simulink model "HITL_Plant_top"  (R2026a)
settings: Solver=VariableStepAuto  StopTime=inf
undefined symbols (not defined in the file): airspeed, ddx, ddy, ddz, dx, dy, dz, fractalcoef, gpsFreq, heartbeatFreq, m_to_mm, ms_to_cms, p, Payload, pitch, q, r, roll, SampleTime, uT_to_gauss, X, Y, yaw, Z
libraries: uavmavlinklib x9, simulink x4, px4MAVLinkBridgelib x2, aerolibatmos2 x1, sensorgpslib x1, robotcorelib x1, mspsensorlib x1
settings Model: DataDictionary=VTOLDynamicsData.sldd  SimulationMode=accelerator  Creator=The MathWorks, Inc.  LastModifiedBy=The MathWorks, Inc.
settings RTWCC: LargeConstantGeneration=WriteOnlyDNNConstantsToDataFiles

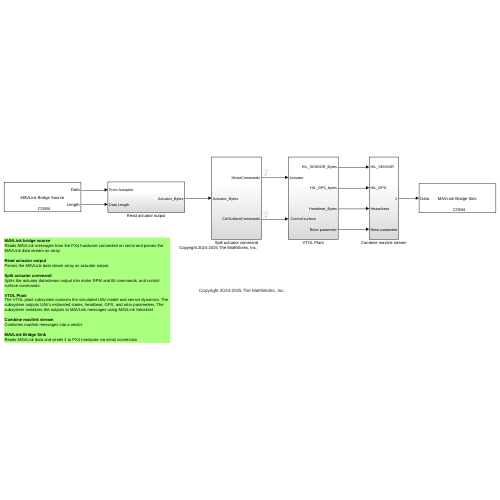
[thumbnail: Simulink's stored preview of the top-level diagram]
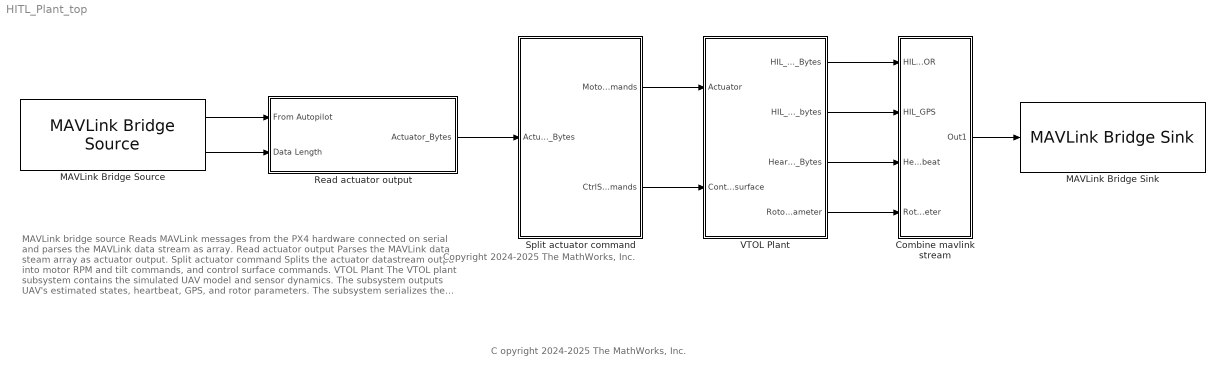
== system HITL_Plant_top ==
  note: MAVLink bridge source
      | Reads MAVLink messages from the PX4 hardware connected on serial and parses the MAVLink data stream as array.
      |
      | Read actuator output
      | Parses the MAVLink data steam array as actuator output.
      |
      | Split actuator command
      | Splits the actuator datastream output into motor RPM and tilt commands, and control surface commands.
      |
      | VTOL Plant
      | The VTOL plant subsystem contains the simulated UAV model and sensor dynamics. The subsystem outputs UAV's estimated states, heartbeat, GPS, and rotor parameters. The subsystem serializes the outputs to MAVLink messages using MAVLink Serializer
      |
      | Combine mavlink stream
      | Combines mavlink messages into a vector
      |
      | MAVLink Bridge Sink
      | Reads MAVLink data and sends it to PX4 hardware via serial connection
  note: C opyright 2024-2025 The MathWorks, Inc.
  note: Copyright 2024-2025 The MathWorks, Inc.
  Combine mavlink stream : Subsystem
  MAVLink Bridge Sink : px4MAVLinkBridgelib/MAVLink Bridge Sink  PixhawkSerialPorttemp=Specify manually  PixhawkSerialPortManually=COM4  FieldTable={ 'UDP', '127.0.0.1', '14550'; 'UDP', '127.0.0.1', '25000' }
  MAVLink Bridge Source : px4MAVLinkBridgelib/MAVLink Bridge Source  PixhawkSerialPorttemp=Specify manually  PixhawkSerialPortManually=COM4  dataLength=MAVLink_Input_Read_Size  FieldTable={ 'UDP', '127.0.0.1', '14550'; 'UDP', '127.0.0.1', '25000' }  SampleTime=SampleTime
  Read actuator output : Subsystem
  Split actuator command : Subsystem
  VTOL Plant : Subsystem
  wires:
  MAVLink Bridge Source/1 -> Read actuator output/1(From Autopilot)
  MAVLink Bridge Source/2 -> Read actuator output/2(Data Length)
  Read actuator output/1(Actuator_Bytes) -> Split actuator command/1(Actuator_Bytes)
  Split actuator command/1(MotorCommands) -> VTOL Plant/1(Actuator)
  Split actuator command/2(CtrlSurfaceCommands) -> VTOL Plant/2(" Control surface")
  Combine mavlink stream/1(Out1) -> MAVLink Bridge Sink/1
  VTOL Plant/2(HIL_GPS_bytes) -> Combine mavlink stream/2(HIL_GPS)
  VTOL Plant/3(Heartbeat_Bytes) -> Combine mavlink stream/3(Heaartbeat)
  VTOL Plant/4(Rotor parameter) -> Combine mavlink stream/4(Rotor parameter)
  VTOL Plant/1(HIL_SENSOR_Bytes) -> Combine mavlink stream/1(HIL_SENSOR)

== system HITL_Plant_top/Combine mavlink stream ==
  HIL_SENSOR : Inport
  HIL_GPS : Inport  Port=2
  Heaartbeat : Inport  Port=3
  Rotor parameter : Inport  Port=4
  Mux : Mux
  Out1 : Outport
  wires:
  Mux/1 -> Out1/1
  HIL_SENSOR/1 -> Mux/1
  HIL_GPS/1 -> Mux/2
  Heaartbeat/1 -> Mux/3
  Rotor parameter/1 -> Mux/4

== system HITL_Plant_top/Read actuator output ==
  From Autopilot : Inport
  Data Length : Inport  Port=2
  Constant : Constant  SampleTime=SampleTime
  Constant1 : Constant  Value=0  OutDataTypeStr=uint8  SampleTime=SampleTime
  Data Type Conversion : DataTypeConversion  OutDataTypeStr=double  SaturateOnIntegerOverflow=off  RndMeth=Floor
  Mux : Mux  Inputs=2
  Reshape : Reshape
  Selector : Selector  InputPortWidth=MAVLink_Input_Read_Size  IndexOptions=Starting and ending indices (port)  Indices=[1 3]  OutputSizes=1
  Switch : Switch  Criteria=u2 > Threshold  SaturateOnIntegerOverflow=off  InputSameDT=off
  Actuator_Bytes : Outport
  wires:
  Mux/1 -> Selector/2
  Constant/1 -> Mux/1
  Data Length/1 -> Data Type Conversion/1
  From Autopilot/1 -> Selector/1
  Switch/1 -> Reshape/1
  Selector/1 -> Switch/1
  Data Type Conversion/1 -> Switch/2, Mux/2
  Reshape/1 -> Actuator_Bytes/1
  Constant1/1 -> Switch/3

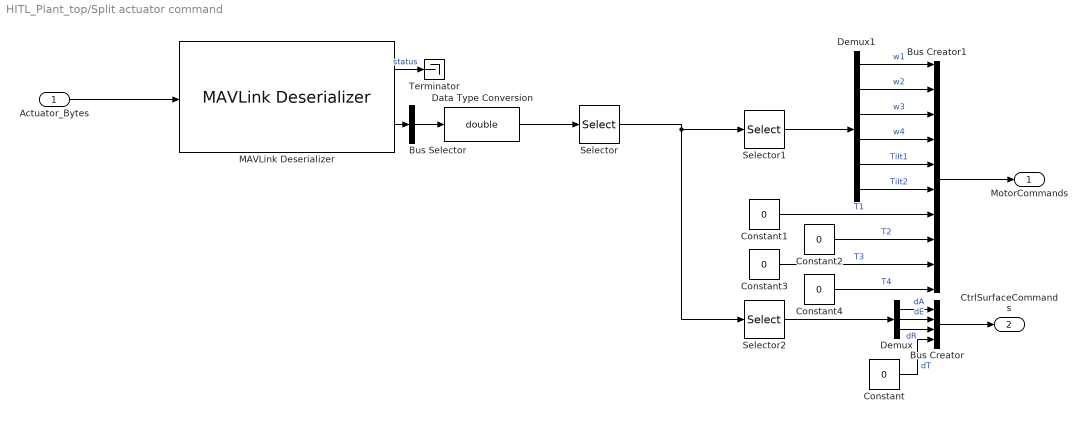
== system HITL_Plant_top/Split actuator command ==
  Actuator_Bytes : Inport
  Bus Creator : BusCreator  Inputs=4  OutDataTypeStr=Bus: FixedWingCtrlBus
  Bus Creator1 : BusCreator  Inputs=10  OutDataTypeStr=Bus: RotorCtrlBus
  Bus Selector : BusSelector  OutputSignals=Payload.controls  OutputAsBus=on
  Constant{,1..4} (5 alike) : Constant  Value=0
  Data Type Conversion : DataTypeConversion  OutDataTypeStr=double  SaturateOnIntegerOverflow=off  RndMeth=Floor
  Demux : Demux  Outputs=3
  Demux1 : Demux  Outputs=6
  MAVLink Deserializer : uavmavlinklib/MAVLink Deserializer  dialectSource=Select from standard MAVLink dialects  dialect=common.xml  dialectCustom=common.xml  version=2  messageType=HIL_ACTUATOR_CONTROLS  inputDataLength=off  SystemIDFilter=off  systemID=1  ComponentIDFilter=off  componentID=1  queueMsg=off  queueMsgSize=50  dropNum=off
  Selector : Selector  InputPortWidth=16  IndexOptions=Index vector (dialog)  Indices=[1:9]  OutputSizes=1
  Selector1 : Selector  InputPortWidth=9  IndexOptions=Index vector (dialog)  Indices=[1:6]  OutputSizes=1
  Selector2 : Selector  InputPortWidth=9  IndexOptions=Index vector (dialog)  Indices=[7:9]  OutputSizes=1
  Terminator : Terminator
  MotorCommands : Outport
  CtrlSurfaceCommands : Outport  Port=2
  wires:
  Actuator_Bytes/1 -> MAVLink Deserializer/1
  Bus Creator1/1 -> MotorCommands/1
  Demux/1 -> Bus Creator/1  "dA"
  Demux1/6 -> Bus Creator1/6  "Tilt2"
  Data Type Conversion/1 -> Selector/1
  Bus Creator/1 -> CtrlSurfaceCommands/1
  Demux1/1 -> Bus Creator1/1  "w1"
  Demux/2 -> Bus Creator/2  "dE"
  MAVLink Deserializer/2 -> Bus Selector/1
  Demux1/2 -> Bus Creator1/2  "w2"
  Demux1/5 -> Bus Creator1/5  "Tilt1"
  MAVLink Deserializer/1 -> Terminator/1  "status"
  Selector2/1 -> Demux/1
  Demux/3 -> Bus Creator/3  "dR"
  Demux1/3 -> Bus Creator1/3  "w3"
  Demux1/4 -> Bus Creator1/4  "w4"
  Bus Selector/1 -> Data Type Conversion/1
  Selector1/1 -> Demux1/1
  Selector/1 -> Selector2/1, Selector1/1
  Constant/1 -> Bus Creator/4  "dT"
  Constant1/1 -> Bus Creator1/7  "T1"
  Constant2/1 -> Bus Creator1/8  "T2"
  Constant3/1 -> Bus Creator1/9  "T3"
  Constant4/1 -> Bus Creator1/10  "T4"

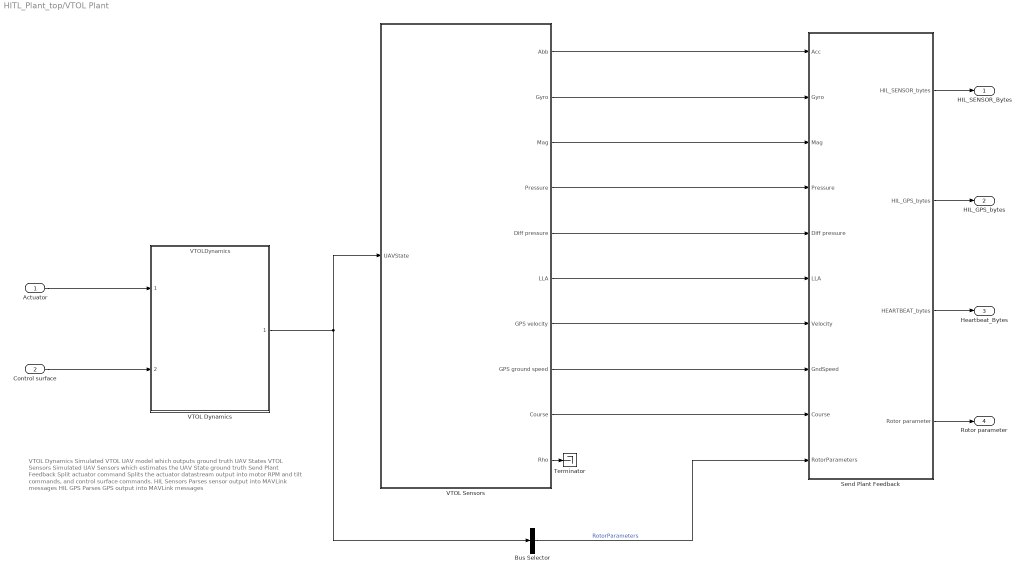
== system HITL_Plant_top/VTOL Plant ==
  note: VTOL Dynamics
      | Simulated VTOL UAV model which outputs ground truth UAV States
      |
      | VTOL Sensors
      | Simulated UAV Sensors which estimates the UAV State ground truth
      |
      | Send Plant Feedback
      | Split actuator command
      | Splits the actuator datastream output into motor RPM and tilt commands, and control surface commands.
      |
      | HIL Sensors
      | Parses sensor output into MAVLink messages
      |
      | HIL GPS
      | Parses GPS output into MAVLink messages
  Actuator : Inport
  " Control surface" : Inport  Port=2
  Bus Selector : BusSelector  OutputSignals=RotorParameters  OutputAsBus=on
  Send Plant Feedback : Subsystem
  Terminator : Terminator
  VTOL Dynamics : ModelReference  ModelNameDialog=VTOLDynamics  SimulationMode=Normal  ModelReferenceVersion=4.0
  VTOL Sensors : Subsystem
  HIL_SENSOR_Bytes : Outport
  HIL_GPS_bytes : Outport  Port=2
  Heartbeat_Bytes : Outport  Port=3
  Rotor parameter : Outport  Port=4
  wires:
  Actuator/1 -> VTOL Dynamics/1
  " Control surface"/1 -> VTOL Dynamics/2
  VTOL Dynamics/1 -> Bus Selector/1, VTOL Sensors/1(UAVState)
  VTOL Sensors/10(Rho) -> Terminator/1
  VTOL Sensors/1(Abb) -> Send Plant Feedback/1(Acc)
  VTOL Sensors/2(Gyro) -> Send Plant Feedback/2(Gyro)
  VTOL Sensors/3(Mag) -> Send Plant Feedback/3(Mag)
  VTOL Sensors/4(Pressure) -> Send Plant Feedback/4(Pressure)
  VTOL Sensors/5(Diff pressure) -> Send Plant Feedback/5(Diff pressure)
  VTOL Sensors/6(LLA) -> Send Plant Feedback/6(LLA)
  VTOL Sensors/7(GPS velocity) -> Send Plant Feedback/7(Velocity)
  VTOL Sensors/8(GPS ground speed) -> Send Plant Feedback/8(GndSpeed)
  VTOL Sensors/9(Course) -> Send Plant Feedback/9(Course)
  Bus Selector/1 -> Send Plant Feedback/10(RotorParameters)  "RotorParameters"
  Send Plant Feedback/1(HIL_SENSOR_bytes) -> HIL_SENSOR_Bytes/1
  Send Plant Feedback/2(HIL_GPS_bytes) -> HIL_GPS_bytes/1
  Send Plant Feedback/3(HEARTBEAT_bytes) -> Heartbeat_Bytes/1
  Send Plant Feedback/4(Rotor parameter) -> Rotor parameter/1

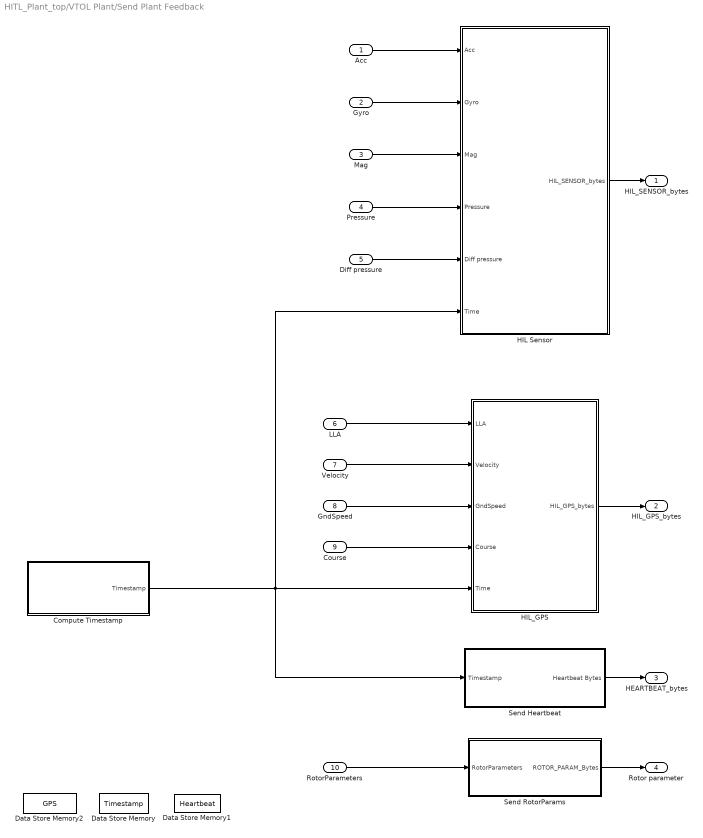
== system HITL_Plant_top/VTOL Plant/Send Plant Feedback ==
  Acc : Inport
  Gyro : Inport  Port=2
  Mag : Inport  Port=3
  Pressure : Inport  Port=4
  Diff pressure : Inport  Port=5
  LLA : Inport  Port=6
  Velocity : Inport  Port=7
  GndSpeed : Inport  Port=8
  Course : Inport  Port=9
  RotorParameters : Inport  Port=10
  Compute Timestamp : Subsystem  Priority=1
  Data Store Memory : DataStoreMemory  DataStoreName=Timestamp  WriteAfterWriteMsg=warning  ShowAdditionalParam=off
  Data Store Memory1 : DataStoreMemory  DataStoreName=Heartbeat  WriteAfterWriteMsg=warning  ShowAdditionalParam=off
  Data Store Memory2 : DataStoreMemory  DataStoreName=GPS  WriteAfterWriteMsg=warning  ShowAdditionalParam=off
  HIL Sensor : Subsystem  Priority=2
  HIL_GPS : Subsystem  Priority=3
  Send Heartbeat : Subsystem  Priority=4
  Send RotorParams : Subsystem  Priority=5
  HIL_SENSOR_bytes : Outport
  HIL_GPS_bytes : Outport  Port=2
  HEARTBEAT_bytes : Outport  Port=3
  Rotor parameter : Outport  Port=4
  wires:
  Send Heartbeat/1(Heartbeat Bytes) -> HEARTBEAT_bytes/1
  RotorParameters/1 -> Send RotorParams/1(RotorParameters)
  Mag/1 -> HIL Sensor/3(Mag)
  Send RotorParams/1(ROTOR_PARAM_Bytes) -> Rotor parameter/1
  Course/1 -> HIL_GPS/4(Course)
  Velocity/1 -> HIL_GPS/2(Velocity)
  Gyro/1 -> HIL Sensor/2(Gyro)
  GndSpeed/1 -> HIL_GPS/3(GndSpeed)
  Pressure/1 -> HIL Sensor/4(Pressure)
  HIL Sensor/1(HIL_SENSOR_bytes) -> HIL_SENSOR_bytes/1
  Acc/1 -> HIL Sensor/1(Acc)
  LLA/1 -> HIL_GPS/1(LLA)
  Diff pressure/1 -> HIL Sensor/5(Diff pressure)
  HIL_GPS/1(HIL_GPS_bytes) -> HIL_GPS_bytes/1
  Compute Timestamp/1(Timestamp) -> Send Heartbeat/1(Timestamp), HIL Sensor/6(Time), HIL_GPS/5(Time)

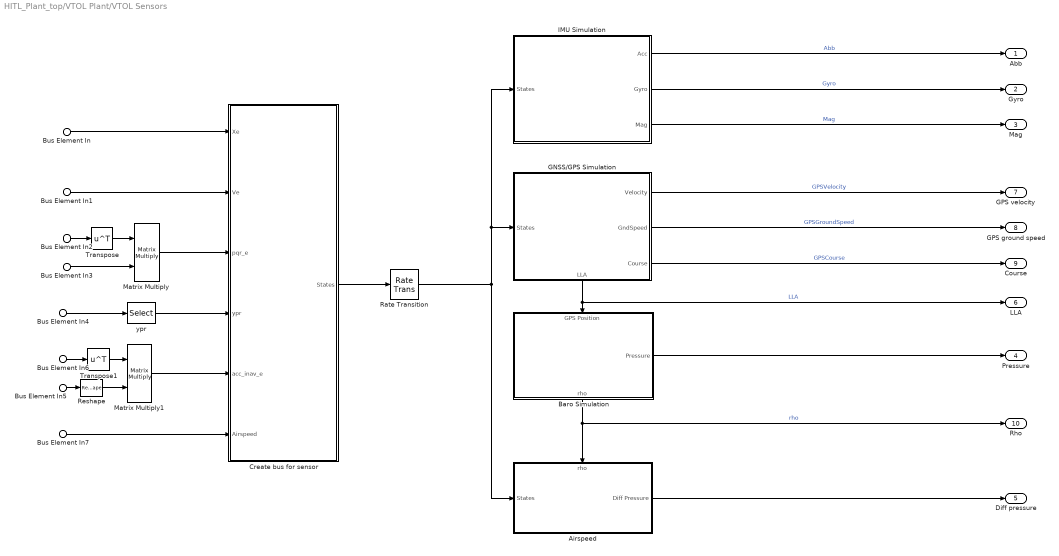
== system HITL_Plant_top/VTOL Plant/VTOL Sensors ==
  Bus Element In : Inport  PortName=UAVState  Element=Xe
  Bus Element In1 : Inport  PortName=UAVState  Element=Ve
  Bus Element In2 : Inport  PortName=UAVState  Element=DCMbe
  Bus Element In6 : Inport  PortName=UAVState  Element=DCMbe
  Bus Element In3 : Inport  PortName=UAVState  Element=pqr
  Bus Element In4 : Inport  PortName=UAVState  Element=Euler
  Bus Element In5 : Inport  PortName=UAVState  Element=Abe
  Bus Element In7 : Inport  PortName=UAVState  Element=airspeed
  " Baro Simulation" : Subsystem
      settings: PortSchema="{\"entries\":[{\"content\":{\"sides\":[{\"content\":{},\"type\":\"ConnectorPlacement.EquallySpacedRectSide\",\"uuid\":\"7ecc8b21-8f8f-4144-826a-6b68e30dbf7d\"},{\"content\":{\"connectorIds\":[\"Out1\"],\"side\":\"RIGHT\"},\"type\":\"ConnectorPlacement.EquallySpacedRectSide\",\"uuid\":\"81a1dd55-8330-4386-9921-36c0eb60d526\"},{\"content\":{\"connectorIds\":[\"In1\"],\"side\":\"TOP\"},\"type\":\"ConnectorPlacement.EquallySpacedRectSide\",\"uuid\":\"b99caff5-b40d-407d-b30e-35210c1aee1d\"},{\"content\":{\"connectorIds\":[\"Out2\"],\"side\":\"BOTTOM\"},\"type\":\"ConnectorPlacement.EquallySpacedRectSide\",\"uuid\":\"18bfda3d-4fab-4e61-9ebc-e384e51de306\"}]},\"type\":\"ConnectorPlacement.EquallySpacedConnector\",\"uuid\":\"17ab4e96-b761-4c62-a0bb-ab626dac3eaa\"}],\"packageUris\":[\"http://schema.mathworks.com/mf0/Connector/R2020b\"],\"version\":\"1.0\"}"
  Airspeed : Subsystem
      settings: PortSchema="{\"entries\":[{\"content\":{\"sides\":[{\"content\":{\"connectorIds\":[\"In1\"]},\"type\":\"ConnectorPlacement.EquallySpacedRectSide\",\"uuid\":\"3559b1c7-c417-4679-ba34-14fe3bb5fa42\"},{\"content\":{\"connectorIds\":[\"Out1\"],\"side\":\"RIGHT\"},\"type\":\"ConnectorPlacement.EquallySpacedRectSide\",\"uuid\":\"d110bf6e-f7b9-4997-879d-ad1455a93ca8\"},{\"content\":{\"connectorIds\":[\"In2\"],\"side\":\"TOP\"},\"type\":\"ConnectorPlacement.EquallySpacedRectSide\",\"uuid\":\"260deb0e-8534-463c-a5c1-f7f48450a244\"}]},\"type\":\"ConnectorPlacement.EquallySpacedConnector\",\"uuid\":\"5cf6edc7-4001-4afc-aecb-2748ffe02c01\"}],\"packageUris\":[\"http://schema.mathworks.com/mf0/Connector/R2020b\"],\"version\":\"1.0\"}"
  Create bus for sensor : Subsystem
  GNSS/GPS Simulation : Subsystem
      settings: PortSchema="{\"entries\":[{\"content\":{\"sides\":[{\"content\":{\"connectorIds\":[\"In1\"]},\"type\":\"ConnectorPlacement.EquallySpacedRectSide\",\"uuid\":\"4934e8ff-5d4b-4e11-968d-c23bd62383a0\"},{\"content\":{\"connectorIds\":[\"Out1\",\"Out2\",\"Out3\"],\"side\":\"RIGHT\"},\"type\":\"ConnectorPlacement.EquallySpacedRectSide\",\"uuid\":\"9ec8bc0a-2d3c-4dca-835c-010ac29b6ebc\"},{\"content\":{\"connectorIds\":[],\"side\":\"TOP\"},\"type\":\"ConnectorPlacement.EquallySpacedRectSide\",\"uuid\":\"04f09eb4-1bd9-450e-b951-47054bdd92ad\"},{\"content\":{\"connectorIds\":[\"Out4\"],\"side\":\"BOTTOM\"},\"type\":\"ConnectorPlacement.EquallySpacedRectSide\",\"uuid\":\"54bba437-6d13-4ada-8e8d-b8e04495ee78\"}]},\"type\":\"ConnectorPlacement.EquallySpacedConnector\",\"uuid\":\"9a5920cf-a58d-4c98-839b-fbac94edbe7e\"}],\"packageUris\":[\"http://schema.mathworks.com/mf0/Connector/R2020b\"],\"version\":\"1.0\"}"
  IMU Simulation : Subsystem
  Matrix Multiply : Product  Multiplication=Matrix(*)
  Matrix Multiply1 : Product  Multiplication=Matrix(*)
  Rate Transition : RateTransition  OutPortSampleTime=SampleTime
  Reshape : Reshape  OutputDimensionality=Column vector (2-D)
  Transpose : Math  Operator=transpose
  Transpose1 : Math  Operator=transpose
  ypr : Selector  InputPortWidth=3  IndexOptions=Index vector (dialog)  Indices=[3 2 1]  OutputSizes=1
  Abb : Outport
  Gyro : Outport  Port=2
  Mag : Outport  Port=3
  Pressure : Outport  Port=4
  Diff pressure : Outport  Port=5
  LLA : Outport  Port=6
  GPS velocity : Outport  Port=7
  GPS ground speed : Outport  Port=8
  Course : Outport  Port=9
  Rho : Outport  Port=10
  wires:
  Bus Element In2/1 -> Transpose/1
  Transpose/1 -> Matrix Multiply/1
  Bus Element In3/1 -> Matrix Multiply/2
  Bus Element In4/1 -> ypr/1
  Transpose1/1 -> Matrix Multiply1/1
  Bus Element In5/1 -> Reshape/1
  Bus Element In6/1 -> Transpose1/1
  Bus Element In/1 -> Create bus for sensor/1(Xe)
  GNSS/GPS Simulation/3(Course) -> Course/1  "GPSCourse"
  Airspeed/1(Diff Pressure) -> Diff pressure/1
  IMU Simulation/1(Acc) -> Abb/1  "Abb"
  Rate Transition/1 -> IMU Simulation/1(States), GNSS/GPS Simulation/1(States), Airspeed/1(States)
  GNSS/GPS Simulation/2(GndSpeed) -> GPS ground speed/1  "GPSGroundSpeed"
  " Baro Simulation"/1(Pressure) -> Pressure/1
  IMU Simulation/3(Mag) -> Mag/1  "Mag"
  GNSS/GPS Simulation/4(LLA) -> LLA/1, " Baro Simulation"/1(GPS Position)  "LLA"
  " Baro Simulation"/2(rho) -> Rho/1, Airspeed/2(rho)  "rho"
  GNSS/GPS Simulation/1(Velocity) -> GPS velocity/1  "GPSVelocity"
  IMU Simulation/2(Gyro) -> Gyro/1  "Gyro"
  Create bus for sensor/1(States) -> Rate Transition/1
  Bus Element In1/1 -> Create bus for sensor/2(Ve)
  Matrix Multiply/1 -> Create bus for sensor/3(pqr_e)
  ypr/1 -> Create bus for sensor/4(ypr)
  Matrix Multiply1/1 -> Create bus for sensor/5(acc_inav_e)
  Bus Element In7/1 -> Create bus for sensor/6(Airspeed)
  Reshape/1 -> Matrix Multiply1/2

== system HITL_Plant_top/VTOL Plant/Send Plant Feedback/Compute Timestamp ==
  Add : Sum
  Constant : Constant  Value=SampleTime*1e6  OutDataTypeStr=uint64  SampleTime=SampleTime
  Data Store Read : DataStoreRead  DataStoreName=Timestamp  SampleTime=SampleTime  IndexOptions=Index vector (dialog)  Indices=1  OutputSizes=1
  Data Store Write : DataStoreWrite  DataStoreName=Timestamp  SampleTime=SampleTime  IndexOptions=Index vector (dialog)  Indices=1  OutputSizes=1
  Timestamp : Outport
  wires:
  Data Store Read/1 -> Add/1
  Add/1 -> Timestamp/1, Data Store Write/1  "Timestamp"
  Constant/1 -> Add/2

== system HITL_Plant_top/VTOL Plant/Send Plant Feedback/HIL Sensor ==
  Acc : Inport
  Gyro : Inport  Port=2
  Mag : Inport  Port=3
  Pressure : Inport  Port=4
  Diff pressure : Inport  Port=5
  Time : Inport  Port=6
  HIL_SENSOR Creation subsystem : Subsystem
  MAVLink Serializer1 : uavmavlinklib/MAVLink Serializer  dialectSource=Select from standard MAVLink dialects  dialect=common.xml  dialectCustom=common.xml  version=2  messageType=HIL_SENSOR
  Rate Transition : RateTransition  OutPortSampleTime=SampleTime
  Terminator : Terminator
  HIL_SENSOR_bytes : Outport
  wires:
  Acc/1 -> HIL_SENSOR Creation subsystem/1(Acc)
  Gyro/1 -> HIL_SENSOR Creation subsystem/2(Gyro)
  Mag/1 -> HIL_SENSOR Creation subsystem/3(Mag)
  Pressure/1 -> HIL_SENSOR Creation subsystem/4(Pressure)
  Diff pressure/1 -> HIL_SENSOR Creation subsystem/5(Diff Pressure)
  Rate Transition/1 -> MAVLink Serializer1/1
  MAVLink Serializer1/2 -> Terminator/1
  MAVLink Serializer1/1 -> HIL_SENSOR_bytes/1
  HIL_SENSOR Creation subsystem/1(HIL Sensor) -> Rate Transition/1
  Time/1 -> HIL_SENSOR Creation subsystem/6(Time)

== system HITL_Plant_top/VTOL Plant/Send Plant Feedback/HIL_GPS ==
  LLA : Inport
  Velocity : Inport  Port=2
  GndSpeed : Inport  Port=3
  Course : Inport  Port=4
  Time : Inport  Port=5
  GPS : Subsystem
  GPS Serialization : Subsystem
  HIL_GPS_bytes : Outport
  wires:
  LLA/1 -> GPS Serialization/1(LLA)
  Velocity/1 -> GPS Serialization/2(Velocity)
  GndSpeed/1 -> GPS Serialization/3(GndSpeed)
  Course/1 -> GPS Serialization/4(Course)
  Time/1 -> GPS/2(Timestamp), GPS Serialization/5(Time)
  GPS Serialization/1(GPS Bytes) -> GPS/1(GPS Bytes)
  GPS/1(GPS Value) -> HIL_GPS_bytes/1
  GPS/2(Update GPS) -> GPS Serialization/Enable

== system HITL_Plant_top/VTOL Plant/Send Plant Feedback/Send Heartbeat ==
  Timestamp : Inport
  GPS : Subsystem
  Heartbeat_Serialization : Subsystem
  Heartbeat Bytes : Outport
  wires:
  Heartbeat_Serialization/1(Heartbeat) -> GPS/1(Heartbeat Bytes)
  Timestamp/1 -> GPS/2(Timestamp)
  GPS/1(Update Heartbeat) -> Heartbeat_Serialization/Enable
  GPS/2(Heartbeat Value) -> Heartbeat Bytes/1

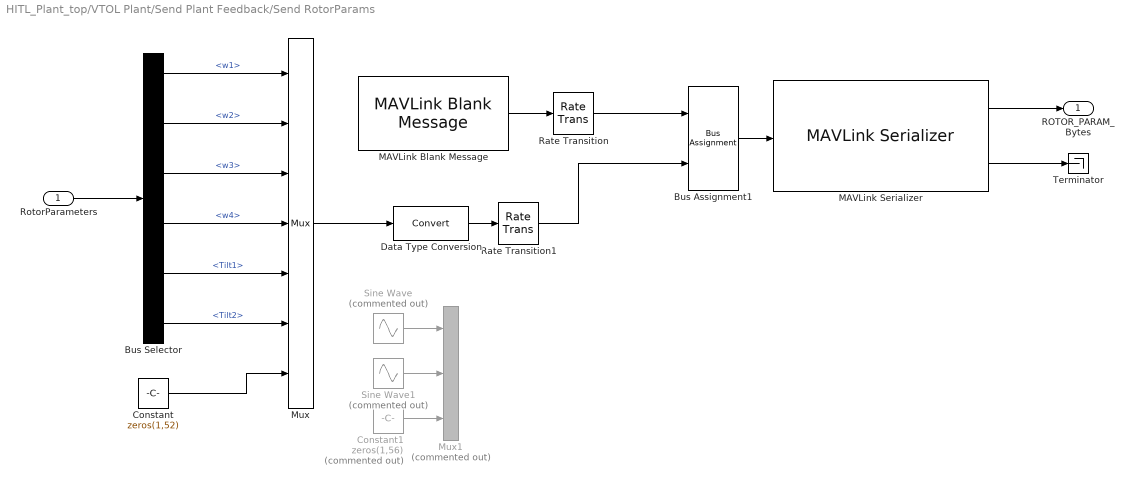
== system HITL_Plant_top/VTOL Plant/Send Plant Feedback/Send RotorParams ==
  RotorParameters : Inport
  Bus Assignment1 : BusAssignment  AssignedSignals=Payload.data
  Bus Selector : BusSelector  OutputSignals=w1,w2,w3,w4,Tilt1,Tilt2
  Constant : Constant  Value=zeros(1,52)  SampleTime=-1
  Constant1 : Constant  Commented=on  Value=zeros(1,56)  SampleTime=-1
  Data Type Conversion : DataTypeConversion  SaturateOnIntegerOverflow=off  RndMeth=Floor
  MAVLink Blank Message : uavmavlinklib/MAVLink Blank Message  dialectSource=Select from standard MAVLink dialects  dialect=common.xml  dialectCustom=common.xml  version=2  messageType=DEBUG_FLOAT_ARRAY  SystemID=1  ComponentID=1  SampleTime=-1
  MAVLink Serializer : uavmavlinklib/MAVLink Serializer  dialectSource=Select from standard MAVLink dialects  dialect=common.xml  dialectCustom=common.xml  version=2  messageType=DEBUG_FLOAT_ARRAY
  Mux : Mux  Inputs=7
  Mux1 : Mux  Commented=on  Inputs=3
  Rate Transition : RateTransition  OutPortSampleTime=SampleTime
  Rate Transition1 : RateTransition  OutPortSampleTime=SampleTime
  Sine Wave : Sin  Commented=on  SampleTime=0
  Sine Wave1 : Sin  Commented=on  Amplitude=2  SampleTime=0
  Terminator : Terminator
  ROTOR_PARAM_Bytes : Outport
  wires:
  RotorParameters/1 -> Bus Selector/1
  Bus Selector/1 -> Mux/1  "<w1>"
  Bus Selector/2 -> Mux/2  "<w2>"
  Bus Selector/3 -> Mux/3  "<w3>"
  Bus Selector/4 -> Mux/4  "<w4>"
  Bus Selector/5 -> Mux/5  "<Tilt1>"
  Bus Selector/6 -> Mux/6  "<Tilt2>"
  Constant/1 -> Mux/7
  MAVLink Blank Message/1 -> Rate Transition/1
  Bus Assignment1/1 -> MAVLink Serializer/1
  MAVLink Serializer/1 -> ROTOR_PARAM_Bytes/1
  MAVLink Serializer/2 -> Terminator/1
  Data Type Conversion/1 -> Rate Transition1/1
  Sine Wave/1 -> Mux1/1
  Sine Wave1/1 -> Mux1/2
  Constant1/1 -> Mux1/3
  Mux/1 -> Data Type Conversion/1
  Rate Transition/1 -> Bus Assignment1/1
  Rate Transition1/1 -> Bus Assignment1/2

== system HITL_Plant_top/VTOL Plant/VTOL Sensors/ Baro Simulation ==
  GPS Position : Inport
  Extract Altitude : Selector  InputPortWidth=3  IndexOptions=Index vector (dialog)  Indices=[3]  OutputSizes=1
  Gain1 : Gain  Gain=1/1000
  Gain2 : Gain  Gain=1000
  Lapse Rate Model : aerolibatmos2/ISA Atmosphere Model  useExtended=off  action=Warning  custom=on  viscosityOut=off  g=9.80665  gamma=1.4  R=287.0531  L=0.0065  h_trop=11000  h_strat=20000  rho0=1.225  P0=101325  T0=288.15  h0=0  S=110.4  Tref=273.15  muref=1.716e-5
  Random Number1 : RandomNumber  Variance=10  Seed=10  SampleTime=SampleTime
  Sum1 : Sum  Inputs=|++
  Terminator : Terminator
  Terminator1 : Terminator
  Pressure : Outport
  rho : Outport  Port=2
  wires:
  Random Number1/1 -> Sum1/2  "Pressure_noise"
  GPS Position/1 -> Extract Altitude/1
  Gain1/1 -> Lapse Rate Model/1
  Extract Altitude/1 -> Gain2/1
  Gain2/1 -> Sum1/1
  Sum1/1 -> Gain1/1
  Lapse Rate Model/3 -> Pressure/1
  Lapse Rate Model/1 -> Terminator/1
  Lapse Rate Model/4 -> rho/1
  Lapse Rate Model/2 -> Terminator1/1

== system HITL_Plant_top/VTOL Plant/VTOL Sensors/Airspeed ==
  In Bus Element : Inport  PortName=States  Element=airspeed
  rho : Inport  Port=2
  Constant : Constant  Value=0.5  SampleTime=-1
  Constant1 : Constant  Value=0  SampleTime=-1
  Max : MinMax  Function=max  Inputs=2
  Product : Product  Inputs=3
  Random Number1 : RandomNumber  Variance=0.1  Seed=545  SampleTime=SampleTime
  Square : Math  Operator=square
  Sum : Sum  Inputs=|++
  Diff Pressure : Outport
  wires:
  Constant1/1 -> Max/2
  Sum/1 -> Max/1
  Max/1 -> Diff Pressure/1
  Random Number1/1 -> Sum/2  "Pressure_noise"
  Product/1 -> Sum/1
  In Bus Element/1 -> Square/1
  Square/1 -> Product/1
  rho/1 -> Product/2
  Constant/1 -> Product/3

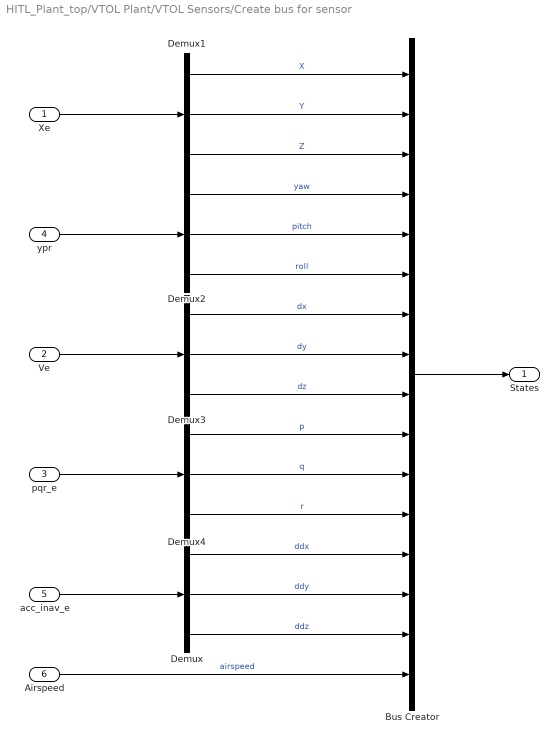
== system HITL_Plant_top/VTOL Plant/VTOL Sensors/Create bus for sensor ==
  Xe : Inport
  Ve : Inport  Port=2
  pqr_e : Inport  Port=3
  ypr : Inport  Port=4
  acc_inav_e : Inport  Port=5
  Airspeed : Inport  Port=6
  Bus Creator : BusCreator  Inputs=X,Y,Z,yaw,pitch,roll,dx,dy,dz,p,q,r,ddx,ddy,ddz,airspeed
  Demux{,1..4} (5 alike) : Demux  Outputs=3
  States : Outport
  wires:
  Xe/1 -> Demux1/1
  Demux3/1 -> Bus Creator/7  "dx"
  Demux1/1 -> Bus Creator/1  "X"
  Demux1/2 -> Bus Creator/2  "Y"
  Demux/2 -> Bus Creator/14  "ddy"
  Demux3/3 -> Bus Creator/9  "dz"
  Bus Creator/1 -> States/1
  Airspeed/1 -> Bus Creator/16  "airspeed"
  Demux2/3 -> Bus Creator/6  "roll"
  Demux/1 -> Bus Creator/13  "ddx"
  Demux2/1 -> Bus Creator/4  "yaw"
  Demux/3 -> Bus Creator/15  "ddz"
  Demux4/3 -> Bus Creator/12  "r"
  Demux3/2 -> Bus Creator/8  "dy"
  Demux4/2 -> Bus Creator/11  "q"
  ypr/1 -> Demux2/1
  acc_inav_e/1 -> Demux/1
  Demux2/2 -> Bus Creator/5  "pitch"
  Ve/1 -> Demux3/1
  Demux1/3 -> Bus Creator/3  "Z"
  pqr_e/1 -> Demux4/1
  Demux4/1 -> Bus Creator/10  "p"

== system HITL_Plant_top/VTOL Plant/VTOL Sensors/GNSS//GPS Simulation ==
  States : Inport
  Bus Selector : BusSelector  OutputSignals=dx,dy,dz  OutputAsBus=on
  Bus Selector1 : BusSelector  OutputSignals=X,Y,Z  OutputAsBus=on
  GPS1 : sensorgpslib/GPS  DispRefFrame=NED  PositionInputFormat=Local  ReferenceLocation=[47.398,8.5456,488]  HorizontalPositionAccuracy=0.005  VerticalPositionAccuracy=0.005  VelocityAccuracy=0.005  DecayFactor=0.99  SeedDouble=68  SimulateUsing=Interpreted execution
  Reshape1 : Reshape  OutputDimensionality=Row vector (2-D)
  Reshape3 : Reshape  OutputDimensionality=Row vector (2-D)
  Velocity : Outport
  GndSpeed : Outport  Port=2
  Course : Outport  Port=3
  LLA : Outport  Port=4
  wires:
  GPS1/4 -> Course/1
  GPS1/3 -> GndSpeed/1
  States/1 -> Bus Selector1/1, Bus Selector/1
  GPS1/2 -> Velocity/1
  Reshape1/1 -> GPS1/2
  Bus Selector/1 -> Reshape1/1
  Bus Selector1/1 -> Reshape3/1
  GPS1/1 -> LLA/1  "lla"
  Reshape3/1 -> GPS1/1

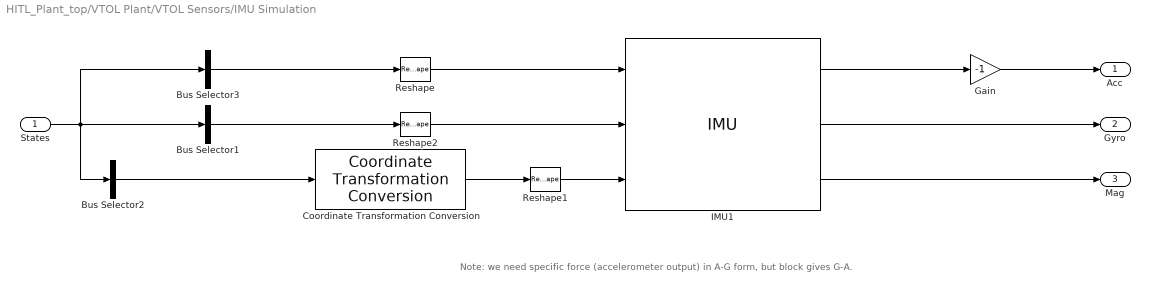
== system HITL_Plant_top/VTOL Plant/VTOL Sensors/IMU Simulation ==
  note: Note:
      | we need specific force (accelerometer output) in A-G form, but block gives G-A.
  States : Inport
  Bus Selector1 : BusSelector  OutputSignals=p,q,r  OutputAsBus=on
  Bus Selector2 : BusSelector  OutputSignals=yaw,pitch,roll  OutputAsBus=on
  Bus Selector3 : BusSelector  OutputSignals=ddx,ddy,ddz  OutputAsBus=on
  Coordinate Transformation Conversion : robotcorelib/Coordinate Transformation Conversion  InputRepresentation=Euler Angles  InputEulerSequence=ZYX  ShowTrVecInputPort=on  OutputRepresentation=Quaternion  OutputEulerSequence=ZYX  ShowTrVecOutputPort=on  SimulateUsing=Code generation
  Gain : Gain  Gain=-1
  IMU1 : mspsensorlib/IMU  DispRefFrame=NED  TemperaturePort=off  Temperature=25  MagneticFieldPort=off  MagneticFieldNED=[21.5 1.16 43.1]  MagneticFieldENU=[ -2.4169, 27.5550, 16.0849 ]  SeedDouble=87254  SimulateUsing=Interpreted execution  AccelParamsMeasurementRange=Inf  AccelParamsResolution=0  AccelParamsConstantBias=[ 0, 0, 0 ]  AccelParamsAxesMisalignment=[ 0, 0, 0 ]  AccelParamsNoiseDensity=0.0003  AccelParamsBiasInstability=[ 0, 0, 0 ]  AccelParamsBiasInstabilityNumerator=fractalcoef().Numerator  AccelParamsBiasInstabilityDenominator=fractalcoef().Denominator  AccelParamsRandomWalk=[ 0, 0, 0 ]  AccelParamsNoiseType=double-sided  AccelParamsTemperatureBias=[ 0, 0, 0 ]  AccelParamsTemperatureScaleFactor=[ 0, 0, 0 ]  GyroParamsMeasurementRange=Inf  GyroParamsResolution=0  GyroParamsConstantBias=[ 0, 0, 0 ]  GyroParamsAxesMisalignment=[ 0, 0, 0 ]  GyroParamsAccelerationBias=0.0001  GyroParamsNoiseDensity=0.01  GyroParamsBiasInstability=[ 0, 0, 0 ]  GyroParamsBiasInstabilityNumerator=fractalcoef().Numerator  GyroParamsBiasInstabilityDenominator=fractalcoef().Denominator  GyroParamsRandomWalk=[ 0, 0, 0 ]  GyroParamsNoiseType=double-sided  GyroParamsTemperatureBias=[ 0, 0, 0 ]  GyroParamsTemperatureScaleFactor=[ 0, 0, 0 ]  MagParamsMeasurementRange=Inf  MagParamsResolution=0  MagParamsConstantBias=[ 0, 0, 0 ]  MagParamsAxesMisalignment=[ 0, 0, 0 ]  MagParamsNoiseDensity=0.0005  MagParamsBiasInstability=[ 0, 0, 0 ]  MagParamsBiasInstabilityNumerator=fractalcoef().Numerator  MagParamsBiasInstabilityDenominator=fractalcoef().Denominator  MagParamsRandomWalk=[ 0, 0, 0 ]  MagParamsNoiseType=double-sided  MagParamsTemperatureBias=[ 0, 0, 0 ]  MagParamsTemperatureScaleFactor=[ 0, 0, 0 ]
  Reshape : Reshape  OutputDimensionality=Row vector (2-D)
  Reshape1 : Reshape  OutputDimensionality=Row vector (2-D)
  Reshape2 : Reshape  OutputDimensionality=Row vector (2-D)
  Acc : Outport
  Gyro : Outport  Port=2
  Mag : Outport  Port=3
  wires:
  Reshape1/1 -> IMU1/3
  Reshape/1 -> IMU1/1
  IMU1/2 -> Gyro/1
  IMU1/3 -> Mag/1
  IMU1/1 -> Gain/1
  Coordinate Transformation Conversion/1 -> Reshape1/1
  States/1 -> Bus Selector3/1, Bus Selector2/1, Bus Selector1/1
  Reshape2/1 -> IMU1/2
  Bus Selector2/1 -> Coordinate Transformation Conversion/1
  Bus Selector1/1 -> Reshape2/1
  Bus Selector3/1 -> Reshape/1
  Gain/1 -> Acc/1

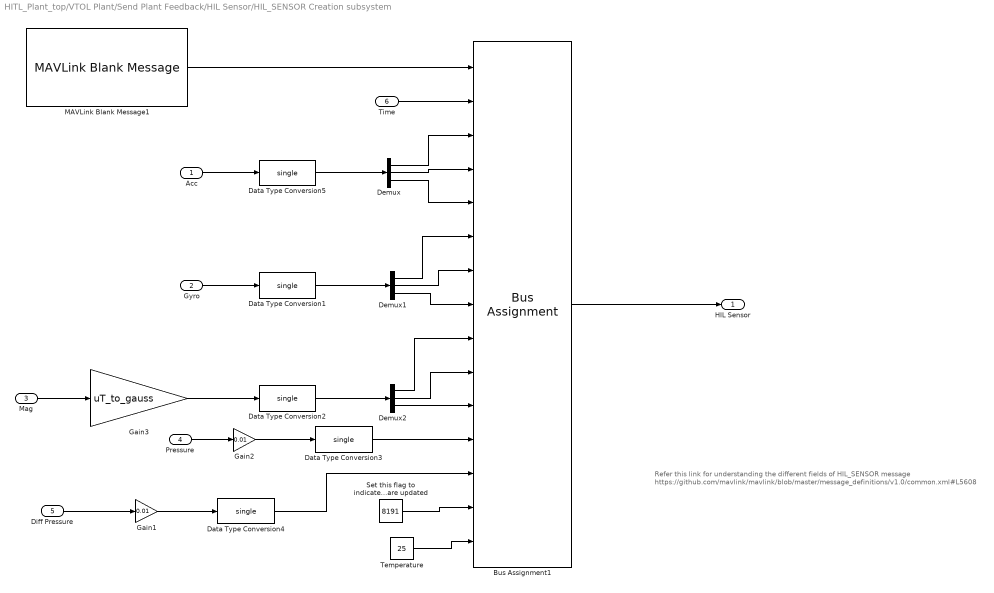
== system HITL_Plant_top/VTOL Plant/Send Plant Feedback/HIL Sensor/HIL_SENSOR Creation subsystem ==
  note: Refer this link for understanding the different fields of HIL_SENSOR message https://github.com/mavlink/mavlink/blob/master/message_definitions/v1.0/common.xml#L5608
  Acc : Inport
  Gyro : Inport  Port=2
  Mag : Inport  Port=3
  Pressure : Inport  Port=4
  Diff Pressure : Inport  Port=5
  Time : Inport  Port=6
  Bus Assignment1 : BusAssignment  AssignedSignals=Payload.time_usec,Payload.xacc,Payload.yacc,Payload.zacc,Payload.xgyro,Payload.ygyro,Payload.zgyro,Payload.xmag,Payload.ymag,Payload.zmag,Payload.abs_pressure,Payload.diff_pressure,Payload.fields_updated,Payload.temperature
  Data Type Conversion{1..5} (5 alike) : DataTypeConversion  OutDataTypeStr=single  SaturateOnIntegerOverflow=off  RndMeth=Floor
  Demux : Demux  Outputs=3
  Demux1 : Demux  Outputs=3
  Demux2 : Demux  Outputs=3
  Gain1 : Gain  Gain=0.01  OutDataTypeStr=single
  Gain2 : Gain  Gain=0.01  OutDataTypeStr=single
  Gain3 : Gain  Gain=uT_to_gauss
  MAVLink Blank Message1 : uavmavlinklib/MAVLink Blank Message  dialectSource=Select from standard MAVLink dialects  dialect=common.xml  dialectCustom=common.xml  version=2  messageType=HIL_SENSOR  SystemID=2  ComponentID=51  SampleTime=-1
  Set this flag to indicate all flags are updated : Constant  Value=8191  OutDataTypeStr=Inherit: Inherit via back propagation  SampleTime=-1
  Temperature : Constant  Value=25  OutDataTypeStr=Inherit: Inherit via back propagation  SampleTime=-1
  HIL Sensor : Outport
  wires:
  Data Type Conversion2/1 -> Demux2/1
  Demux1/1 -> Bus Assignment1/6
  Mag/1 -> Gain3/1
  Demux1/3 -> Bus Assignment1/8
  Data Type Conversion1/1 -> Demux1/1
  Gyro/1 -> Data Type Conversion1/1
  Bus Assignment1/1 -> HIL Sensor/1
  Demux/3 -> Bus Assignment1/5
  Demux2/2 -> Bus Assignment1/10
  Demux2/3 -> Bus Assignment1/11
  Data Type Conversion5/1 -> Demux/1
  Demux/1 -> Bus Assignment1/3
  MAVLink Blank Message1/1 -> Bus Assignment1/1
  Demux2/1 -> Bus Assignment1/9
  Demux/2 -> Bus Assignment1/4
  Demux1/2 -> Bus Assignment1/7
  Acc/1 -> Data Type Conversion5/1
  Data Type Conversion3/1 -> Bus Assignment1/12
  Gain3/1 -> Data Type Conversion2/1
  Set this flag to indicate all flags are updated/1 -> Bus Assignment1/14
  Pressure/1 -> Gain2/1
  Time/1 -> Bus Assignment1/2
  Gain2/1 -> Data Type Conversion3/1
  Temperature/1 -> Bus Assignment1/15
  Diff Pressure/1 -> Gain1/1
  Gain1/1 -> Data Type Conversion4/1
  Data Type Conversion4/1 -> Bus Assignment1/13

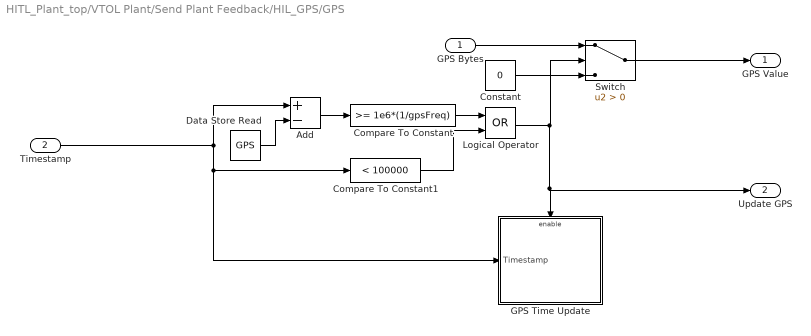
== system HITL_Plant_top/VTOL Plant/Send Plant Feedback/HIL_GPS/GPS ==
  GPS Bytes : Inport
  Timestamp : Inport  Port=2
  Add : Sum  Inputs=+-
  Compare To Constant : simulink/Logic and Bit Operations/Compare To Constant  relop=>=  const=1e6*(1/gpsFreq)  OutDataTypeStr=uint8
  Compare To Constant1 : simulink/Logic and Bit Operations/Compare To Constant  relop=<  const=100000  OutDataTypeStr=boolean
  Constant : Constant  Value=0  OutDataTypeStr=uint8  SampleTime=SampleTime
  Data Store Read : DataStoreRead  DataStoreName=GPS  SampleTime=SampleTime  IndexOptions=Index vector (dialog)  Indices=1  OutputSizes=1
  GPS Time Update : Subsystem
  Logical Operator : Logic  Operator=OR  AllPortsSameDT=off  OutDataTypeStr=boolean
  Switch : Switch  Criteria=u2 > Threshold  SaturateOnIntegerOverflow=off  InputSameDT=off
  GPS Value : Outport
  Update GPS : Outport  Port=2
  wires:
  Timestamp/1 -> GPS Time Update/1(Timestamp), Compare To Constant1/1, Add/1
  Data Store Read/1 -> Add/2
  Add/1 -> Compare To Constant/1
  GPS Bytes/1 -> Switch/1
  Constant/1 -> Switch/3
  Switch/1 -> GPS Value/1
  Compare To Constant/1 -> Logical Operator/1
  Logical Operator/1 -> GPS Time Update/Enable, Update GPS/1, Switch/2
  Compare To Constant1/1 -> Logical Operator/2

== system HITL_Plant_top/VTOL Plant/Send Plant Feedback/HIL_GPS/GPS Serialization ==
  LLA : Inport
  Velocity : Inport  Port=2
  GndSpeed : Inport  Port=3
  Course : Inport  Port=4
  Time : Inport  Port=5
  Enable : EnablePort
  HIL_GPS Subsystem : Subsystem
  MAVLink Serializer3 : uavmavlinklib/MAVLink Serializer  dialectSource=Select from standard MAVLink dialects  dialect=common.xml  dialectCustom=common.xml  version=2  messageType=HIL_GPS
  Rate Transition : RateTransition  OutPortSampleTime=SampleTime
  Terminator : Terminator
  GPS Bytes : Outport
  wires:
  MAVLink Serializer3/1 -> GPS Bytes/1
  Velocity/1 -> HIL_GPS Subsystem/2(Velocity)
  Rate Transition/1 -> MAVLink Serializer3/1
  MAVLink Serializer3/2 -> Terminator/1
  HIL_GPS Subsystem/1(Out1) -> Rate Transition/1
  LLA/1 -> HIL_GPS Subsystem/1(LLA)
  Course/1 -> HIL_GPS Subsystem/4(Course)
  Time/1 -> HIL_GPS Subsystem/5(Time)
  GndSpeed/1 -> HIL_GPS Subsystem/3(GndSpeed)

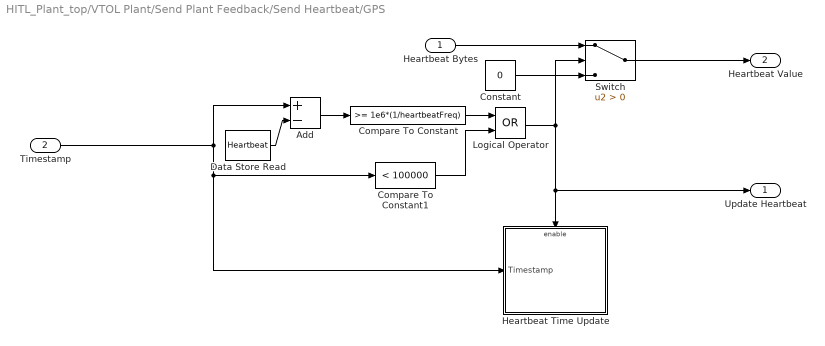
== system HITL_Plant_top/VTOL Plant/Send Plant Feedback/Send Heartbeat/GPS ==
  Heartbeat Bytes : Inport
  Timestamp : Inport  Port=2
  Add : Sum  Inputs=+-
  Compare To Constant : simulink/Logic and Bit Operations/Compare To Constant  relop=>=  const=1e6*(1/heartbeatFreq)  OutDataTypeStr=uint8
  Compare To Constant1 : simulink/Logic and Bit Operations/Compare To Constant  relop=<  const=100000  OutDataTypeStr=boolean
  Constant : Constant  Value=0  OutDataTypeStr=uint8  SampleTime=SampleTime
  Data Store Read : DataStoreRead  DataStoreName=Heartbeat  SampleTime=SampleTime  IndexOptions=Index vector (dialog)  Indices=1  OutputSizes=1
  Heartbeat Time Update : Subsystem
  Logical Operator : Logic  Operator=OR  AllPortsSameDT=off  OutDataTypeStr=boolean
  Switch : Switch  Criteria=u2 > Threshold  SaturateOnIntegerOverflow=off  InputSameDT=off
  Update Heartbeat : Outport
  Heartbeat Value : Outport  Port=2
  wires:
  Timestamp/1 -> Heartbeat Time Update/1(Timestamp), Compare To Constant1/1, Add/1
  Data Store Read/1 -> Add/2
  Add/1 -> Compare To Constant/1
  Heartbeat Bytes/1 -> Switch/1
  Constant/1 -> Switch/3
  Switch/1 -> Heartbeat Value/1
  Compare To Constant1/1 -> Logical Operator/2
  Compare To Constant/1 -> Logical Operator/1
  Logical Operator/1 -> Switch/2, Update Heartbeat/1, Heartbeat Time Update/Enable

== system HITL_Plant_top/VTOL Plant/Send Plant Feedback/Send Heartbeat/Heartbeat_Serialization ==
  Enable : EnablePort
  Bus Assignment : BusAssignment  AssignedSignals=Payload.autopilot,Payload.type
  Constant : Constant  SampleTime=-1
  Constant1 : Constant  Value=12  SampleTime=-1
  Data Type Conversion : DataTypeConversion  OutDataTypeStr=uint8  SaturateOnIntegerOverflow=off  RndMeth=Floor
  Data Type Conversion1 : DataTypeConversion  OutDataTypeStr=uint8  SaturateOnIntegerOverflow=off  RndMeth=Floor
  MAVLink Blank Message : uavmavlinklib/MAVLink Blank Message  dialectSource=Select from standard MAVLink dialects  dialect=common.xml  dialectCustom=common.xml  version=2  messageType=HEARTBEAT  SystemID=2  ComponentID=51  SampleTime=SampleTime
  MAVLink Serializer : uavmavlinklib/MAVLink Serializer  dialectSource=Select from standard MAVLink dialects  dialect=common.xml  dialectCustom=common.xml  version=2  messageType=HEARTBEAT
  Terminator4 : Terminator
  Heartbeat : Outport
  wires:
  Data Type Conversion1/1 -> Bus Assignment/3
  Constant/1 -> Data Type Conversion/1
  Constant1/1 -> Data Type Conversion1/1
  Bus Assignment/1 -> MAVLink Serializer/1
  MAVLink Serializer/2 -> Terminator4/1
  Data Type Conversion/1 -> Bus Assignment/2
  MAVLink Blank Message/1 -> Bus Assignment/1
  MAVLink Serializer/1 -> Heartbeat/1

== system HITL_Plant_top/VTOL Plant/Send Plant Feedback/HIL_GPS/GPS/GPS Time Update ==
  Timestamp : Inport
  Enable : EnablePort
  Update GPS Time : DataStoreWrite  DataStoreName=GPS  IndexOptions=Index vector (dialog)  Indices=1  OutputSizes=1
  wires:
  Timestamp/1 -> Update GPS Time/1

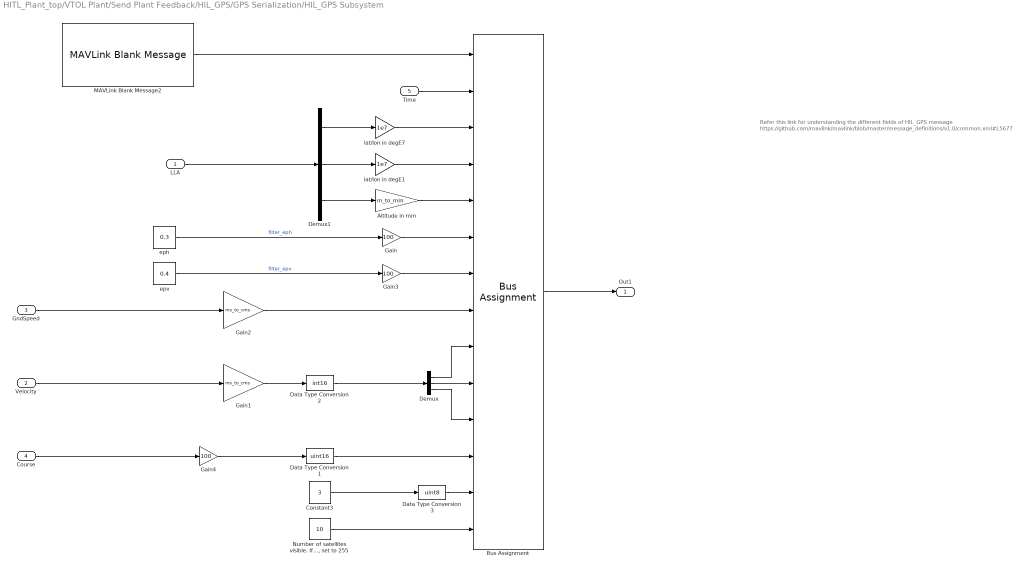
== system HITL_Plant_top/VTOL Plant/Send Plant Feedback/HIL_GPS/GPS Serialization/HIL_GPS Subsystem ==
  note: Refer this link for understanding the different fields of HIL_GPS message https://github.com/mavlink/mavlink/blob/master/message_definitions/v1.0/common.xml#L5677
  LLA : Inport
  Velocity : Inport  Port=2
  GndSpeed : Inport  Port=3
  Course : Inport  Port=4
  Time : Inport  Port=5
  Altitude in mm : Gain  Gain=m_to_mm  OutDataTypeStr=Inherit: Inherit via back propagation
  Bus Assignment : BusAssignment  AssignedSignals=Payload.time_usec,Payload.lat,Payload.lon,Payload.alt,Payload.eph,Payload.epv,Payload.vel,Payload.vn,Payload.ve,Payload.vd,Payload.cog,Payload.fix_type,Payload.satellites_visible
  Constant3 : Constant  Value=3  OutDataTypeStr=Inherit: Inherit via back propagation  SampleTime=-1
  Data Type Conversion1 : DataTypeConversion  OutDataTypeStr=uint16  SaturateOnIntegerOverflow=off  RndMeth=Floor
  Data Type Conversion2 : DataTypeConversion  OutDataTypeStr=int16  SaturateOnIntegerOverflow=off  RndMeth=Floor
  Data Type Conversion3 : DataTypeConversion  OutDataTypeStr=uint8  SaturateOnIntegerOverflow=off  RndMeth=Floor
  Demux : Demux  Outputs=3
  Demux1 : Demux  Outputs=3
  Gain : Gain  Gain=100  OutDataTypeStr=Inherit: Inherit via back propagation
  Gain1 : Gain  Gain=ms_to_cms
  Gain2 : Gain  Gain=ms_to_cms  OutDataTypeStr=uint16
  Gain3 : Gain  Gain=100  OutDataTypeStr=Inherit: Inherit via back propagation
  Gain4 : Gain  Gain=100
  MAVLink Blank Message2 : uavmavlinklib/MAVLink Blank Message  dialectSource=Select from standard MAVLink dialects  dialect=common.xml  dialectCustom=common.xml  version=2  messageType=HIL_GPS  SystemID=2  ComponentID=51  SampleTime=-1
  "Number of satellites visible. If unknown, set to 255" : Constant  Value=10  OutDataTypeStr=Inherit: Inherit via back propagation  SampleTime=-1
  eph : Constant  Value=0.3  SampleTime=-1
  epv : Constant  Value=0.4  SampleTime=-1
  lat/lon in degE1 : Gain  Gain=1e7  OutDataTypeStr=Inherit: Inherit via back propagation
  lat/lon in degE7 : Gain  Gain=1e7  OutDataTypeStr=Inherit: Inherit via back propagation
  Out1 : Outport
  wires:
  Gain2/1 -> Bus Assignment/8
  lat/lon in degE7/1 -> Bus Assignment/3
  Demux1/1 -> lat/lon in degE7/1
  Demux/3 -> Bus Assignment/11
  MAVLink Blank Message2/1 -> Bus Assignment/1
  Gain1/1 -> Data Type Conversion2/1
  Demux1/3 -> Altitude in mm/1
  Demux1/2 -> lat/lon in degE1/1
  Demux/1 -> Bus Assignment/9
  lat/lon in degE1/1 -> Bus Assignment/4
  Altitude in mm/1 -> Bus Assignment/5
  Data Type Conversion2/1 -> Demux/1
  Demux/2 -> Bus Assignment/10
  Gain/1 -> Bus Assignment/6
  Gain3/1 -> Bus Assignment/7
  GndSpeed/1 -> Gain2/1
  Velocity/1 -> Gain1/1
  Course/1 -> Gain4/1
  Data Type Conversion1/1 -> Bus Assignment/12
  eph/1 -> Gain/1  "filter_eph"
  epv/1 -> Gain3/1  "filter_epv"
  Data Type Conversion3/1 -> Bus Assignment/13
  Gain4/1 -> Data Type Conversion1/1
  Time/1 -> Bus Assignment/2
  LLA/1 -> Demux1/1
  Bus Assignment/1 -> Out1/1
  Constant3/1 -> Data Type Conversion3/1
  "Number of satellites visible. If unknown, set to 255"/1 -> Bus Assignment/14

== system HITL_Plant_top/VTOL Plant/Send Plant Feedback/Send Heartbeat/GPS/Heartbeat Time Update ==
  Timestamp : Inport
  Enable : EnablePort
  Update Heartbeat Time : DataStoreWrite  DataStoreName=Heartbeat  IndexOptions=Index vector (dialog)  Indices=1  OutputSizes=1
  wires:
  Timestamp/1 -> Update Heartbeat Time/1
